simulink model "sysArch"  (R2025a)
settings: Solver=VariableStepAuto  StartTime=0.0  StopTime=10.0  RelTol=1e-3
settings Model: Creator=aidan  LastModifiedBy=aidan

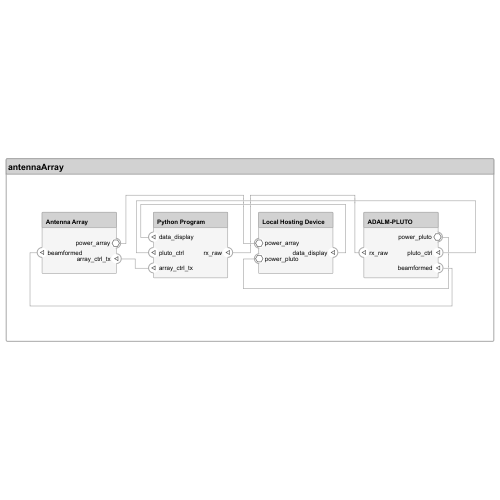
[thumbnail: Simulink's stored preview of the top-level diagram]
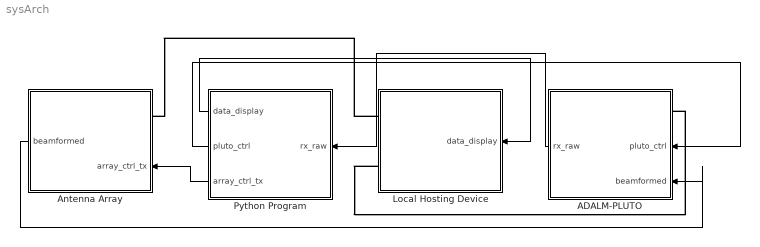
== system sysArch ==
  ADALM-PLUTO : Subsystem
      settings: PortSchema="{\"entries\":[{\"content\":{\"headerSize\":26,\"margin\":15,\"minimumSpacing\":25,\"sides\":[{\"content\":{\"connectorIds\":[\"Out1\"]},\"type\":\"ConnectorPlacement.EquallySpacedRectSide\",\"uuid\":\"82cd1861-f582-407e-baf2-1313af35079b\"},{\"content\":{\"connectorIds\":[\"RConn1\",\"In1\",\"In2\"],\"side\":\"RIGHT\"},\"type\":\"ConnectorPlacement.EquallySpacedRectSide\",\"uuid\":\"76c44748-c661-4c79-81a7-401c7c764583\"},{\"content\":{\"side\":\"TOP\"},\"type\":\"ConnectorPlacement.EquallySpacedRectSide\",\"uuid\":\"b3bece90-4550-4988-b515-d3acc4205134\"}]},\"type\":\"ConnectorPlacement.EquallySpacedConnector\",\"uuid\":\"29cc3884-0762-4fbf-8cc3-4c82f7c056a0\"}],\"packageUris\":[\"http://schema.mathworks.com/mf0/Connector/R2020b\"],\"version\":\"1.0\"}"
  Antenna Array : Subsystem
      settings: PortSchema="{\"entries\":[{\"content\":{\"headerSize\":26,\"margin\":15,\"minimumSpacing\":25,\"sides\":[{\"content\":{\"connectorIds\":[\"Out1\"]},\"type\":\"ConnectorPlacement.EquallySpacedRectSide\",\"uuid\":\"82cd1861-f582-407e-baf2-1313af35079b\"},{\"content\":{\"connectorIds\":[\"RConn1\",\"In1\"],\"side\":\"RIGHT\"},\"type\":\"ConnectorPlacement.EquallySpacedRectSide\",\"uuid\":\"76c44748-c661-4c79-81a7-401c7c764583\"},{\"content\":{\"side\":\"TOP\"},\"type\":\"ConnectorPlacement.EquallySpacedRectSide\",\"uuid\":\"b3bece90-4550-4988-b515-d3acc4205134\"}]},\"type\":\"ConnectorPlacement.EquallySpacedConnector\",\"uuid\":\"29cc3884-0762-4fbf-8cc3-4c82f7c056a0\"}],\"packageUris\":[\"http://schema.mathworks.com/mf0/Connector/R2020b\"],\"version\":\"1.0\"}"
  Local Hosting Device : Subsystem
      settings: PortSchema="{\"entries\":[{\"content\":{\"headerSize\":26,\"margin\":15,\"minimumSpacing\":25,\"sides\":[{\"content\":{\"connectorIds\":[\"LConn1\",\"LConn2\"]},\"type\":\"ConnectorPlacement.EquallySpacedRectSide\",\"uuid\":\"82cd1861-f582-407e-baf2-1313af35079b\"},{\"content\":{\"connectorIds\":[\"In1\"],\"side\":\"RIGHT\"},\"type\":\"ConnectorPlacement.EquallySpacedRectSide\",\"uuid\":\"76c44748-c661-4c79-81a7-401c7c764583\"},{\"content\":{\"side\":\"TOP\"},\"type\":\"ConnectorPlacement.EquallySpacedRectSide\",\"uuid\":\"b3bece90-4550-4988-b515-d3acc4205134\"}]},\"type\":\"ConnectorPlacement.EquallySpacedConnector\",\"uuid\":\"29cc3884-0762-4fbf-8cc3-4c82f7c056a0\"}],\"packageUris\":[\"http://schema.mathworks.com/mf0/Connector/R2020b\"],\"version\":\"1.0\"}"
  Python Program : Subsystem
      settings: PortSchema="{\"entries\":[{\"content\":{\"headerSize\":26,\"margin\":15,\"minimumSpacing\":25,\"sides\":[{\"content\":{\"connectorIds\":[\"Out1\",\"Out2\",\"Out3\"]},\"type\":\"ConnectorPlacement.EquallySpacedRectSide\",\"uuid\":\"82cd1861-f582-407e-baf2-1313af35079b\"},{\"content\":{\"connectorIds\":[\"In1\"],\"side\":\"RIGHT\"},\"type\":\"ConnectorPlacement.EquallySpacedRectSide\",\"uuid\":\"76c44748-c661-4c79-81a7-401c7c764583\"},{\"content\":{\"side\":\"TOP\"},\"type\":\"ConnectorPlacement.EquallySpacedRectSide\",\"uuid\":\"b3bece90-4550-4988-b515-d3acc4205134\"}]},\"type\":\"ConnectorPlacement.EquallySpacedConnector\",\"uuid\":\"29cc3884-0762-4fbf-8cc3-4c82f7c056a0\"}],\"packageUris\":[\"http://schema.mathworks.com/mf0/Connector/R2020b\"],\"version\":\"1.0\"}"
  wires:
  Python Program/1(data_display) -> Local Hosting Device/1(data_display)
  ADALM-PLUTO/1(rx_raw) -> Python Program/1(rx_raw)
  Python Program/2(pluto_ctrl) -> ADALM-PLUTO/1(pluto_ctrl)
  Python Program/3(array_ctrl_tx) -> Antenna Array/1(array_ctrl_tx)
  Antenna Array/1(beamformed) -> ADALM-PLUTO/2(beamformed)
  connections:
  Local Hosting Device/LConn2 -- ADALM-PLUTO/RConn1
  Local Hosting Device/LConn1 -- Antenna Array/RConn1

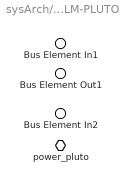
== system sysArch/ADALM-PLUTO ==
  Bus Element In1 : Inport  PortName=pluto_ctrl
  Bus Element In2 : Inport  Port=2  PortName=beamformed
  power_pluto : PMIOPort  Side=Right
  Bus Element Out1 : Outport  PortName=rx_raw

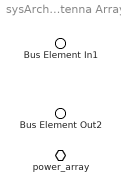
== system sysArch/Antenna Array ==
  Bus Element In1 : Inport  PortName=array_ctrl_tx
  power_array : PMIOPort  Side=Right
  Bus Element Out2 : Outport  PortName=beamformed

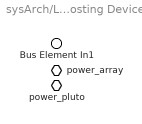
== system sysArch/Local Hosting Device ==
  Bus Element In1 : Inport  PortName=data_display
  power_array : PMIOPort  Side=Left
  power_pluto : PMIOPort  Port=2  Side=Left

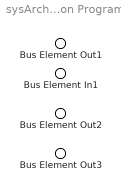
== system sysArch/Python Program ==
  Bus Element In1 : Inport  PortName=rx_raw
  Bus Element Out1 : Outport  PortName=data_display
  Bus Element Out2 : Outport  Port=2  PortName=pluto_ctrl
  Bus Element Out3 : Outport  Port=3  PortName=array_ctrl_tx
